simulink subsystem "MCU"  (R2022a)
settings: Solver=VariableStepAuto  StartTime=0.0  StopTime=10.0  RelTol=1e-3
settings Model: Creator=mmarq  LastModifiedBy=mmarq

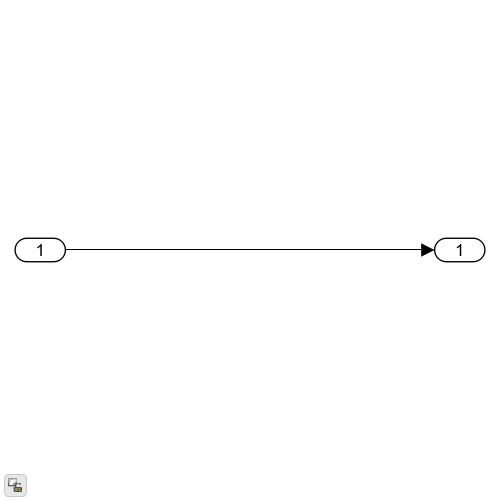
[thumbnail: Simulink's stored preview of the top-level diagram]
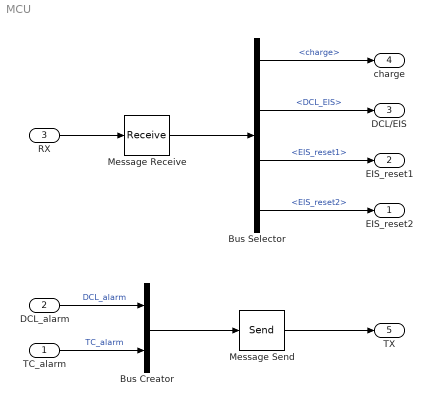
== system MCU ==
  TC_alarm : Inport
  DCL_alarm : Inport  Port=2
  RX : Inport  Port=3  OutDataTypeStr=Bus: MCUCmd
  Bus Creator : BusCreator  Inputs=2  OutDataTypeStr=Bus: MCUData  NonVirtualBus=on
  Bus Selector : BusSelector  OutputSignals=charge,DCL_EIS,EIS_reset1,EIS_reset2
  Message Receive : Receive  InputPortMessageModes=m  UseInternalQueue=off  QueueOverwriting=on  QueueLength=1
  Message Send : Send  OutputPortMessageModes=m
  EIS_reset2 : Outport
  EIS_reset1 : Outport  Port=2
  DCL/EIS : Outport  Port=3
  charge : Outport  Port=4
  TX : Outport  Port=5  OutDataTypeStr=Bus: MCUData
  wires:
  RX/1 -> Message Receive/1
  Message Receive/1 -> Bus Selector/1
  Bus Selector/2 -> DCL/EIS/1  "<DCL_EIS>"
  Bus Selector/1 -> charge/1  "<charge>"
  Bus Selector/4 -> EIS_reset2/1  "<EIS_reset2>"
  Bus Selector/3 -> EIS_reset1/1  "<EIS_reset1>"
  Bus Creator/1 -> Message Send/1
  Message Send/1 -> TX/1
  DCL_alarm/1 -> Bus Creator/1  "DCL_alarm"
  TC_alarm/1 -> Bus Creator/2  "TC_alarm"
